simulink model "eVTOL_System"  (R2024b)
settings: Solver=FixedStepAuto  StartTime=0.0  StopTime=inf  RelTol=1e-3
undefined symbols (not defined in the file): airspeed, Battery, BCE12, BCE_Set_init, BMS_Controller_State, C, Cell10_P, Cell11_P, Cell12_P, Cell13_P, Cell14_P, Cell15_P, Cell16_P, Cell17_P, Cell18_P, Cell19_P, Cell1_N, Cell1_P, Cell20_P, Cell21_P, Cell22_P, Cell23_P, Cell24_P, Cell2_P, Cell3_P, Cell4_P, Cell5_P, Cell6_P, Cell7_P, Cell8_P, Cell9_P, Charging_State, CityMission, control, controlParams, ControlSampleTime, CriticalTiltAngle, currentFactor, CV_Gain, ddx, ddy, ddz, Device_01, Device_02, DiscIntNeverNeededParam, dx, dy, dz, Earth, env, F, F28379D_ADC_MaxCount, F28379D_ADC_Vmax, FixedWingMission, flightState, Foc_Ki_IxTcpu, Foc_Ki_S, Foc_Kp_I, Foc_Kp_S, fractalcoef ... (+68)
libraries: fl_lib x1115, nesl_utility x617, slrealtimeethercatlib x217, simulink x130, canmsglib x101, speedgoatlib_IO611_obsolete x91, slpidlib x49, mcbcontrolslib x44, slrealtimeutilitieslib x35, speedgoatlib_hdlCoder_IO3xx x31, dspstat3 x24, mcbpositiondecoderlib x12
(part 5 of 31)

== system eVTOL_System/Motor Drive/Controller1/Controller_MIL ==
  Iab : Inport
  QAE_MIL_fbk : Inport  Port=2
  EnablePWM : Inport  Port=3
  Closed_Loop_FOC : Inport  Port=4
  Speed_CMD_RPM : Inport  Port=5
  Controller_Parameters : Inport  Port=6
  Bus Creator : BusCreator  Inputs=5
  Bus Selector : BusSelector  OutputSignals=Ia_offset,Ib_offset,Kp_S,Ki_S,Kp_I,Ki_IxTcpu
  Constant : Constant  Value=0  OutDataTypeStr=single  SampleTime=Ts_CPU
  Constant4 : Constant
  Data Type Conversion : DataTypeConversion  SaturateOnIntegerOverflow=off  RndMeth=Floor
  Data Type Conversion1 : DataTypeConversion  OutDataTypeStr=double  SaturateOnIntegerOverflow=off  RndMeth=Floor
  Data Type Conversion2 : DataTypeConversion  OutDataTypeStr=boolean  SaturateOnIntegerOverflow=off  RndMeth=Floor
  Data Type Conversion4 : DataTypeConversion  OutDataTypeStr=boolean  SaturateOnIntegerOverflow=off  RndMeth=Floor
  Data Type Conversion6 : DataTypeConversion  OutDataTypeStr=uint16  RndMeth=Simplest  SaturateOnIntegerOverflow=off
  F28379D ADC : Subsystem
  F28379D Firmware : Subsystem
  IO334 DAC : Subsystem
  Mux : Mux  Inputs=3
  PWM Generation : pwm_cpulib/PWM Generation  f_FPGA=f_FPGA  n_channels=3  sel_scaling=CPU  protection_param=A/B are forced off when A/B are on.  deadband_sec=0  natural_update=At period starts  delay=0  trigger_duration_sec=[1e-6]  trigger_period_start=off  trigger_half_of_the_period=off  trigger_a_on=off  trigger_a_off=off  trigger_b_on=off  trigger_b_off=off  bit_width_pwm_gen=24  invert_a=off  invert_b=off  invert_c=off  showPhaseInput=off
      settings: SourceProductName=PWM CPU Library
  PWM Periods : Constant  Value=[1/PWM_frequency 1/PWM_frequency 1/PWM_frequency]  OutDataTypeStr=double  SampleTime=-1
  Rate Transition1 : RateTransition  OutPortSampleTime=Ts_speed
  Rate Transition12 : RateTransition  OutPortSampleTime=Ts_UI
  Rate Transition{2,4..9} (7 alike) : RateTransition  OutPortSampleTime=Ts_CPU
  Rate Transition3 : RateTransition  OutPortSampleTime=Ts_speed
  bias1 : Constant  OutDataTypeStr=boolean  SampleTime=Ts_CPU
  bias3 : Constant  Value=0  OutDataTypeStr=boolean  SampleTime=Ts_CPU
  Simu_config : Outport
  Controller_fbk : Outport  Port=2
  wires:
  bias1/1 -> Bus Creator/1  "PCIe_RC_or_TTL"
  Bus Creator/1 -> Simu_config/1
  Constant4/1 -> Data Type Conversion6/1
  Data Type Conversion/1 -> Bus Creator/4  "PCIe_PWM_Enable"
  Iab/1 -> IO334 DAC/1(Iab)
  IO334 DAC/1(Iab_IO334DAC) -> F28379D ADC/1(Iab_IO334V)  "IabV"
  F28379D ADC/1(Ia_ADC) -> F28379D Firmware/1(Ia_ADC)
  F28379D ADC/2(Ib_ADC) -> F28379D Firmware/2(Ib_ADC)
  QAE_MIL_fbk/1 -> F28379D Firmware/5(QEP_Position_Count)
  Data Type Conversion6/1 -> F28379D Firmware/6(QEP_Index_Latch)
  Bus Selector/3 -> Rate Transition3/1  "<Kp_S>"
  F28379D Firmware/2(PWM_Enable) -> Data Type Conversion/1
  Data Type Conversion2/1 -> F28379D Firmware/11(EnablePWM)
  Data Type Conversion4/1 -> F28379D Firmware/10(EnClosedLoop)
  Bus Selector/4 -> Rate Transition1/1  "<Ki_S>"
  Closed_Loop_FOC/1 -> Rate Transition4/1
  Controller_Parameters/1 -> Bus Selector/1
  Bus Selector/1 -> Rate Transition5/1  "<Ia_offset>"
  Bus Selector/2 -> Rate Transition6/1  "<Ib_offset>"
  Bus Selector/5 -> Rate Transition8/1  "<Kp_I>"
  Bus Selector/6 -> Rate Transition9/1  "<Ki_IxTcpu>"
  EnablePWM/1 -> Rate Transition7/1
  Mux/1 -> Rate Transition12/1
  F28379D Firmware/3(Fbk_CAN) -> Mux/1
  Speed_CMD_RPM/1 -> Rate Transition2/1
  Rate Transition3/1 -> F28379D Firmware/8(Kp_S)
  Rate Transition1/1 -> F28379D Firmware/9(Ki_S)
  Rate Transition5/1 -> F28379D Firmware/3(IaOffset)
  Rate Transition6/1 -> F28379D Firmware/4(IbOffset)
  Rate Transition4/1 -> Data Type Conversion4/1
  Rate Transition7/1 -> Data Type Conversion2/1
  Rate Transition8/1 -> F28379D Firmware/12(Kp_i)
  Rate Transition9/1 -> F28379D Firmware/13(Ki_ixTcpu)
  Rate Transition12/1 -> Controller_fbk/1
  Constant/1 -> Mux/3
  Rate Transition2/1 -> F28379D Firmware/7(SpdCmdRPM), Mux/2
  bias3/1 -> Bus Creator/5  "PCIe_Protocol"
  PWM Periods/1 -> PWM Generation/1
  PWM Generation/1 -> Bus Creator/2  "PCIe_PWM_Config"
  PWM Generation/2 -> Bus Creator/3  "PCIe_PWM_Runtime"
  Data Type Conversion1/1 -> PWM Generation/2
  F28379D Firmware/1(ModWave) -> Data Type Conversion1/1

== system eVTOL_System/Motor Drive/Controller2/Controller_MIL ==
  Iab : Inport
  QAE_MIL_fbk : Inport  Port=2
  EnablePWM : Inport  Port=3
  Closed_Loop_FOC : Inport  Port=4
  Speed_CMD_RPM : Inport  Port=5
  Controller_Parameters : Inport  Port=6
  Bus Creator : BusCreator  Inputs=5
  Bus Selector : BusSelector  OutputSignals=Ia_offset,Ib_offset,Kp_S,Ki_S,Kp_I,Ki_IxTcpu
  Constant : Constant  Value=0  OutDataTypeStr=single  SampleTime=Ts_CPU
  Constant4 : Constant
  Data Type Conversion : DataTypeConversion  SaturateOnIntegerOverflow=off  RndMeth=Floor
  Data Type Conversion1 : DataTypeConversion  OutDataTypeStr=double  SaturateOnIntegerOverflow=off  RndMeth=Floor
  Data Type Conversion2 : DataTypeConversion  OutDataTypeStr=boolean  SaturateOnIntegerOverflow=off  RndMeth=Floor
  Data Type Conversion4 : DataTypeConversion  OutDataTypeStr=boolean  SaturateOnIntegerOverflow=off  RndMeth=Floor
  Data Type Conversion6 : DataTypeConversion  OutDataTypeStr=uint16  RndMeth=Simplest  SaturateOnIntegerOverflow=off
  F28379D ADC : Subsystem
  F28379D Firmware : Subsystem
  IO334 DAC : Subsystem
  Mux : Mux  Inputs=3
  PWM Generation : pwm_cpulib/PWM Generation  f_FPGA=f_FPGA  n_channels=3  sel_scaling=CPU  protection_param=A/B are forced off when A/B are on.  deadband_sec=0  natural_update=At period starts  delay=0  trigger_duration_sec=[1e-6]  trigger_period_start=off  trigger_half_of_the_period=off  trigger_a_on=off  trigger_a_off=off  trigger_b_on=off  trigger_b_off=off  bit_width_pwm_gen=24  invert_a=off  invert_b=off  invert_c=off  showPhaseInput=off
      settings: SourceProductName=PWM CPU Library
  PWM Periods : Constant  Value=[1/PWM_frequency 1/PWM_frequency 1/PWM_frequency]  OutDataTypeStr=double  SampleTime=-1
  Rate Transition1 : RateTransition  OutPortSampleTime=Ts_speed
  Rate Transition12 : RateTransition  OutPortSampleTime=Ts_UI
  Rate Transition{2,4..9} (7 alike) : RateTransition  OutPortSampleTime=Ts_CPU
  Rate Transition3 : RateTransition  OutPortSampleTime=Ts_speed
  bias1 : Constant  OutDataTypeStr=boolean  SampleTime=Ts_CPU
  bias3 : Constant  Value=0  OutDataTypeStr=boolean  SampleTime=Ts_CPU
  Simu_config : Outport
  Controller_fbk : Outport  Port=2
  wires:
  bias1/1 -> Bus Creator/1  "PCIe_RC_or_TTL"
  Bus Creator/1 -> Simu_config/1
  Constant4/1 -> Data Type Conversion6/1
  Data Type Conversion/1 -> Bus Creator/4  "PCIe_PWM_Enable"
  Iab/1 -> IO334 DAC/1(Iab)
  IO334 DAC/1(Iab_IO334DAC) -> F28379D ADC/1(Iab_IO334V)  "IabV"
  F28379D ADC/1(Ia_ADC) -> F28379D Firmware/1(Ia_ADC)
  F28379D ADC/2(Ib_ADC) -> F28379D Firmware/2(Ib_ADC)
  QAE_MIL_fbk/1 -> F28379D Firmware/5(QEP_Position_Count)
  Data Type Conversion6/1 -> F28379D Firmware/6(QEP_Index_Latch)
  Bus Selector/3 -> Rate Transition3/1  "<Kp_S>"
  F28379D Firmware/2(PWM_Enable) -> Data Type Conversion/1
  Data Type Conversion2/1 -> F28379D Firmware/11(EnablePWM)
  Data Type Conversion4/1 -> F28379D Firmware/10(EnClosedLoop)
  Bus Selector/4 -> Rate Transition1/1  "<Ki_S>"
  Closed_Loop_FOC/1 -> Rate Transition4/1
  Controller_Parameters/1 -> Bus Selector/1
  Bus Selector/1 -> Rate Transition5/1  "<Ia_offset>"
  Bus Selector/2 -> Rate Transition6/1  "<Ib_offset>"
  Bus Selector/5 -> Rate Transition8/1  "<Kp_I>"
  Bus Selector/6 -> Rate Transition9/1  "<Ki_IxTcpu>"
  EnablePWM/1 -> Rate Transition7/1
  Mux/1 -> Rate Transition12/1
  F28379D Firmware/3(Fbk_CAN) -> Mux/1
  Speed_CMD_RPM/1 -> Rate Transition2/1
  Rate Transition3/1 -> F28379D Firmware/8(Kp_S)
  Rate Transition1/1 -> F28379D Firmware/9(Ki_S)
  Rate Transition5/1 -> F28379D Firmware/3(IaOffset)
  Rate Transition6/1 -> F28379D Firmware/4(IbOffset)
  Rate Transition4/1 -> Data Type Conversion4/1
  Rate Transition7/1 -> Data Type Conversion2/1
  Rate Transition8/1 -> F28379D Firmware/12(Kp_i)
  Rate Transition9/1 -> F28379D Firmware/13(Ki_ixTcpu)
  Rate Transition12/1 -> Controller_fbk/1
  Constant/1 -> Mux/3
  Rate Transition2/1 -> F28379D Firmware/7(SpdCmdRPM), Mux/2
  bias3/1 -> Bus Creator/5  "PCIe_Protocol"
  PWM Periods/1 -> PWM Generation/1
  PWM Generation/1 -> Bus Creator/2  "PCIe_PWM_Config"
  PWM Generation/2 -> Bus Creator/3  "PCIe_PWM_Runtime"
  Data Type Conversion1/1 -> PWM Generation/2
  F28379D Firmware/1(ModWave) -> Data Type Conversion1/1

== system eVTOL_System/Motor Drive/Controller3/Controller_MIL ==
  Iab : Inport
  QAE_MIL_fbk : Inport  Port=2
  EnablePWM : Inport  Port=3
  Closed_Loop_FOC : Inport  Port=4
  Speed_CMD_RPM : Inport  Port=5
  Controller_Parameters : Inport  Port=6
  Bus Creator : BusCreator  Inputs=5
  Bus Selector : BusSelector  OutputSignals=Ia_offset,Ib_offset,Kp_S,Ki_S,Kp_I,Ki_IxTcpu
  Constant : Constant  Value=0  OutDataTypeStr=single  SampleTime=Ts_CPU
  Constant4 : Constant
  Data Type Conversion : DataTypeConversion  SaturateOnIntegerOverflow=off  RndMeth=Floor
  Data Type Conversion1 : DataTypeConversion  OutDataTypeStr=double  SaturateOnIntegerOverflow=off  RndMeth=Floor
  Data Type Conversion2 : DataTypeConversion  OutDataTypeStr=boolean  SaturateOnIntegerOverflow=off  RndMeth=Floor
  Data Type Conversion4 : DataTypeConversion  OutDataTypeStr=boolean  SaturateOnIntegerOverflow=off  RndMeth=Floor
  Data Type Conversion6 : DataTypeConversion  OutDataTypeStr=uint16  RndMeth=Simplest  SaturateOnIntegerOverflow=off
  F28379D ADC : Subsystem
  F28379D Firmware : Subsystem
  IO334 DAC : Subsystem
  Mux : Mux  Inputs=3
  PWM Generation : pwm_cpulib/PWM Generation  f_FPGA=f_FPGA  n_channels=3  sel_scaling=CPU  protection_param=A/B are forced off when A/B are on.  deadband_sec=0  natural_update=At period starts  delay=0  trigger_duration_sec=[1e-6]  trigger_period_start=off  trigger_half_of_the_period=off  trigger_a_on=off  trigger_a_off=off  trigger_b_on=off  trigger_b_off=off  bit_width_pwm_gen=24  invert_a=off  invert_b=off  invert_c=off  showPhaseInput=off
      settings: SourceProductName=PWM CPU Library
  PWM Periods : Constant  Value=[1/PWM_frequency 1/PWM_frequency 1/PWM_frequency]  OutDataTypeStr=double  SampleTime=-1
  Rate Transition1 : RateTransition  OutPortSampleTime=Ts_speed
  Rate Transition12 : RateTransition  OutPortSampleTime=Ts_UI
  Rate Transition{2,4..9} (7 alike) : RateTransition  OutPortSampleTime=Ts_CPU
  Rate Transition3 : RateTransition  OutPortSampleTime=Ts_speed
  bias1 : Constant  OutDataTypeStr=boolean  SampleTime=Ts_CPU
  bias3 : Constant  Value=0  OutDataTypeStr=boolean  SampleTime=Ts_CPU
  Simu_config : Outport
  Controller_fbk : Outport  Port=2
  wires:
  bias1/1 -> Bus Creator/1  "PCIe_RC_or_TTL"
  Bus Creator/1 -> Simu_config/1
  Constant4/1 -> Data Type Conversion6/1
  Data Type Conversion/1 -> Bus Creator/4  "PCIe_PWM_Enable"
  Iab/1 -> IO334 DAC/1(Iab)
  IO334 DAC/1(Iab_IO334DAC) -> F28379D ADC/1(Iab_IO334V)  "IabV"
  F28379D ADC/1(Ia_ADC) -> F28379D Firmware/1(Ia_ADC)
  F28379D ADC/2(Ib_ADC) -> F28379D Firmware/2(Ib_ADC)
  QAE_MIL_fbk/1 -> F28379D Firmware/5(QEP_Position_Count)
  Data Type Conversion6/1 -> F28379D Firmware/6(QEP_Index_Latch)
  Bus Selector/3 -> Rate Transition3/1  "<Kp_S>"
  F28379D Firmware/2(PWM_Enable) -> Data Type Conversion/1
  Data Type Conversion2/1 -> F28379D Firmware/11(EnablePWM)
  Data Type Conversion4/1 -> F28379D Firmware/10(EnClosedLoop)
  Bus Selector/4 -> Rate Transition1/1  "<Ki_S>"
  Closed_Loop_FOC/1 -> Rate Transition4/1
  Controller_Parameters/1 -> Bus Selector/1
  Bus Selector/1 -> Rate Transition5/1  "<Ia_offset>"
  Bus Selector/2 -> Rate Transition6/1  "<Ib_offset>"
  Bus Selector/5 -> Rate Transition8/1  "<Kp_I>"
  Bus Selector/6 -> Rate Transition9/1  "<Ki_IxTcpu>"
  EnablePWM/1 -> Rate Transition7/1
  Mux/1 -> Rate Transition12/1
  F28379D Firmware/3(Fbk_CAN) -> Mux/1
  Speed_CMD_RPM/1 -> Rate Transition2/1
  Rate Transition3/1 -> F28379D Firmware/8(Kp_S)
  Rate Transition1/1 -> F28379D Firmware/9(Ki_S)
  Rate Transition5/1 -> F28379D Firmware/3(IaOffset)
  Rate Transition6/1 -> F28379D Firmware/4(IbOffset)
  Rate Transition4/1 -> Data Type Conversion4/1
  Rate Transition7/1 -> Data Type Conversion2/1
  Rate Transition8/1 -> F28379D Firmware/12(Kp_i)
  Rate Transition9/1 -> F28379D Firmware/13(Ki_ixTcpu)
  Rate Transition12/1 -> Controller_fbk/1
  Constant/1 -> Mux/3
  Rate Transition2/1 -> F28379D Firmware/7(SpdCmdRPM), Mux/2
  bias3/1 -> Bus Creator/5  "PCIe_Protocol"
  PWM Periods/1 -> PWM Generation/1
  PWM Generation/1 -> Bus Creator/2  "PCIe_PWM_Config"
  PWM Generation/2 -> Bus Creator/3  "PCIe_PWM_Runtime"
  Data Type Conversion1/1 -> PWM Generation/2
  F28379D Firmware/1(ModWave) -> Data Type Conversion1/1

== system eVTOL_System/Motor Drive/Three-Phase PMSM Drive/PMSM and average inverter ==
  Simu_config : Inport
  V_dc : Inport  Port=2
  Fault : Inport  Port=3
  LdTrq/Spd : Inport  Port=4
  Bus Selector : BusSelector  OutputSignals=PCIe_PWM_Runtime
  Demux : Demux  Outputs=3
  Encoder Simulation : Subsystem
  Idc : Subsystem
  Ideal Inverter : Subsystem
  PMSM : Subsystem
  PMSM HDL Configuration1 : mcbhdlplantlib/PMSM Configuration  portConfig=Torque  Trq_N_mode=0  Ts=Ts_CPU  Pp=7  Rs=0.293  Ld=0.000279  Lq=0.000279  lambda_pm=0.005  J=8.35e-5  B=0.00535  f=0.0065
  Runtime to DC : Subsystem
  Selec Angle1 : Selector  InputPortWidth=14  IndexOptions=Index vector (dialog)  Indices=[10]  OutputSizes=1
  Terminator : Terminator
  Terminator1 : Terminator
  Terminator2 : Terminator
  Ia : Outport
  Ib : Outport  Port=2
  Ic : Outport  Port=3
  Motor_Spd : Outport  Port=4
  Motor_Angle : Outport  Port=5
  QAE_Pos_C : Outport  Port=6
  tag scope: Idc1=global
  wires:
  PMSM/4(RotorMechSpd) -> Motor_Spd/1
  Demux/2 -> Ib/1
  Selec Angle1/1 -> Motor_Angle/1, Encoder Simulation/1(Theta_m)
  Demux/3 -> Ic/1
  LdTrq/Spd/1 -> PMSM/3(LdTrq / Spd)
  PMSM/2(PhaseCurr) -> Demux/1
  Demux/1 -> Idc/1(In1), Ia/1
  Ideal Inverter/1(Vabc) -> PMSM/2(PhaseVolt abc)
  V_dc/1 -> Ideal Inverter/1(V_DC)
  Simu_config/1 -> Bus Selector/1
  Fault/1 -> Terminator/1
  Encoder Simulation/1(QEP_Position_Count) -> QAE_Pos_C/1
  PMSM/3(Torque) -> Terminator1/1
  PMSM/5(RotorElecAngle) -> Terminator2/1
  PMSM/1(Info) -> Selec Angle1/1
  Bus Selector/1 -> Runtime to DC/1(PWM_Runtime)  "<PCIe_PWM_Runtime>"
  Runtime to DC/1(Duty Cycle abc) -> Ideal Inverter/2(Duty Cycle abc)
  PMSM HDL Configuration1/1 -> PMSM/1(Config)
  Idc/1(Out1) -> [Idc1]

== system eVTOL_System/Motor Drive/Three-Phase PMSM Drive/PMSM and inverter with switching dynamics ==
  Simu_config : Inport
  V_dc : Inport  Port=2
  Fault : Inport  Port=3
  LdTrq/Spd : Inport  Port=4
  Bus Selector : BusSelector  OutputSignals=PCIe_RC_or_TTL,PCIe_PWM_Config,PCIe_PWM_Runtime,PCIe_PWM_Enable,PCIe_Protocol
  DAC Config : Subsystem
  Encoder Simulation : Subsystem
  Idc : Subsystem
  Motor Connection : Constant  OutDataTypeStr=boolean
  PMSM HDL Configuration : mcbhdlplantlib/PMSM Configuration  portConfig=Torque  Trq_N_mode=0  Ts=Ts_UI  Pp=Maxon_645604_Np  Rs=Maxon_645604_Rs  Ld=Maxon_645604_Ld  Lq=Maxon_645604_Lq  lambda_pm=Maxon_645604_lambda_pm  J=Maxon_645604_J  B=Maxon_645604_ViscousF*100  f=Maxon_645604_StaticF
  PMSM_3P2L_Inverter_Plant_TBR : Subsystem
      mask Display: disp('Plant Bitstream Block')
  Quadrature Encoder : quadrature_cpulib/Quadrature Encoder  FPGA_freq=f_FPGA  n_channels=[1]  sel_scaling=FPGA  useSpeed=off  usePosition=on  numOfSlots=Maxon_Mile_Nslits  sigAswitchOn=[180]  sigBswitchOff=[90]  sigBswitchOn=[270]  sigAdismissEn=off  sigAdismissSingle=on  sigAdismissHigh=on  sigBdismissEn=off  sigBdismissSingle=on  sigBdismissHigh=on
      settings: SourceProductName=Quadrature CPU Library
  Resolver Encoder : resolver_cpulib/Resolver Encoder  Ts=Ts_UI  ts_resolver=ts_FPGA_mdl  n_channels=1  sel_scaling=FPGA  useSpeed=on  usePosition=off  pole_pairs=1  gain_dynamic=off  gainVector=[1, 1, 1, 1]  offset_dynamic=off  offsetVector=[0, 0, 0, 0]  exct_freq=2  angle_offset=0  exct_amplitude=10  position_init_enb=off  rotor_position=90  int_exct_enb=on  exct_out_enb=on  phase_delay=0  time_step_delay=0  adcRange=2.5  dacRange=2.5
      settings: SourceProductName=Resolver CPU Library
  Terminator{21,32..34,40..41,45..46} (8 alike) : Terminator
  Ia : Outport
  Ib : Outport  Port=2
  Ic : Outport  Port=3
  Motor_Spd : Outport  Port=4
  Motor_Angle : Outport  Port=5
  QAE_Pos_C : Outport  Port=6
  tag scope: Idc1=global
  wires:
  PMSM_3P2L_Inverter_Plant_TBR/10(PCIe_Rsvl_excitation_neg) -> Terminator33/1
  DAC Config/1(I_DAC_gain) -> PMSM_3P2L_Inverter_Plant_TBR/13(PCIe_Iabc_DAC_gain)
  DAC Config/3(DAC_reset) -> PMSM_3P2L_Inverter_Plant_TBR/15(PCIe_DAC_reset)
  PMSM_3P2L_Inverter_Plant_TBR/7(PCIe_Motor_ElecAngle) -> Terminator21/1
  PMSM_3P2L_Inverter_Plant_TBR/12(PCIe_Rsvl_cos_neg) -> Terminator41/1
  PMSM_3P2L_Inverter_Plant_TBR/13(PCIe_Resolver_Out) -> Terminator40/1
  V_dc/1 -> PMSM_3P2L_Inverter_Plant_TBR/6(PCIe_V_dc)
  PMSM_3P2L_Inverter_Plant_TBR/8(PCIe_Motor_Trq) -> Terminator46/1
  Resolver Encoder/1 -> PMSM_3P2L_Inverter_Plant_TBR/12(PCIe_Resolver_Config)
  PMSM_3P2L_Inverter_Plant_TBR/4(PCIe_Idc) -> Terminator45/1
  Quadrature Encoder/1 -> PMSM_3P2L_Inverter_Plant_TBR/11(PCIe_QAE_Config)
  Motor Connection/1 -> PMSM_3P2L_Inverter_Plant_TBR/10(PCIe_Motor_Connection)
  PMSM_3P2L_Inverter_Plant_TBR/9(PCIe_Rsvl_excitation_pos) -> Terminator32/1
  Fault/1 -> PMSM_3P2L_Inverter_Plant_TBR/7(PCIe_Fault)
  PMSM_3P2L_Inverter_Plant_TBR/11(PCIe_Rsvl_sin_neg) -> Terminator34/1
  DAC Config/2(I_DAC_Current) -> PMSM_3P2L_Inverter_Plant_TBR/14(PCIe_Iabc_DAC_bias)
  PMSM HDL Configuration/1 -> PMSM_3P2L_Inverter_Plant_TBR/9(PCIe_Motor_Config)
  Simu_config/1 -> Bus Selector/1
  Bus Selector/4 -> PMSM_3P2L_Inverter_Plant_TBR/4(PCIe_PWM_Enable)  "<PCIe_PWM_Enable>"
  Bus Selector/5 -> PMSM_3P2L_Inverter_Plant_TBR/5(PCIe_Protocol)  "<PCIe_Protocol>"
  Bus Selector/1 -> PMSM_3P2L_Inverter_Plant_TBR/1(PCIe_RC_or_TTL)  "<PCIe_RC_or_TTL>"
  LdTrq/Spd/1 -> PMSM_3P2L_Inverter_Plant_TBR/8(PCIe_LdTrq/Spd)
  PMSM_3P2L_Inverter_Plant_TBR/3(PCIe_Ic) -> Ic/1
  PMSM_3P2L_Inverter_Plant_TBR/6(PCIe_Motor_Angle) -> Motor_Angle/1, Encoder Simulation/1(Theta_m)
  PMSM_3P2L_Inverter_Plant_TBR/5(PCIe_Motor_Spd) -> Motor_Spd/1
  PMSM_3P2L_Inverter_Plant_TBR/2(PCIe_Ib) -> Ib/1
  Encoder Simulation/1(QEP_Position_Count) -> QAE_Pos_C/1
  Bus Selector/3 -> PMSM_3P2L_Inverter_Plant_TBR/3(PCIe_PWM_Runtime)  "<PCIe_PWM_Runtime>"
  Bus Selector/2 -> PMSM_3P2L_Inverter_Plant_TBR/2(PCIe_PWM_Config)  "<PCIe_PWM_Config>"
  Idc/1(Out1) -> [Idc1]
  PMSM_3P2L_Inverter_Plant_TBR/1(PCIe_Ia) -> Idc/1(In1), Ia/1

== system eVTOL_System/Motor Drive/Three-Phase PMSM Drive1/PMSM and average inverter ==
  Simu_config : Inport
  V_dc : Inport  Port=2
  Fault : Inport  Port=3
  LdTrq/Spd : Inport  Port=4
  Bus Selector : BusSelector  OutputSignals=PCIe_PWM_Runtime
  Demux : Demux  Outputs=3
  Encoder Simulation : Subsystem
  Idc : Subsystem
  Ideal Inverter : Subsystem
  PMSM : Subsystem
  PMSM HDL Configuration5 : mcbhdlplantlib/PMSM Configuration  portConfig=Torque  Trq_N_mode=0  Ts=Ts_CPU  Pp=7  Rs=0.293  Ld=0.000279  Lq=0.000279  lambda_pm=0.005  J=8.35e-5  B=0.00535  f=0.0065
  Runtime to DC : Subsystem
  Selec Angle1 : Selector  InputPortWidth=14  IndexOptions=Index vector (dialog)  Indices=[10]  OutputSizes=1
  Terminator : Terminator
  Terminator1 : Terminator
  Terminator2 : Terminator
  Ia : Outport
  Ib : Outport  Port=2
  Ic : Outport  Port=3
  Motor_Spd : Outport  Port=4
  Motor_Angle : Outport  Port=5
  QAE_Pos_C : Outport  Port=6
  tag scope: Idc2=global
  wires:
  PMSM/4(RotorMechSpd) -> Motor_Spd/1
  Demux/2 -> Ib/1
  Selec Angle1/1 -> Motor_Angle/1, Encoder Simulation/1(Theta_m)
  Demux/3 -> Ic/1
  LdTrq/Spd/1 -> PMSM/3(LdTrq / Spd)
  PMSM/2(PhaseCurr) -> Demux/1
  Ideal Inverter/1(Vabc) -> PMSM/2(PhaseVolt abc)
  Simu_config/1 -> Bus Selector/1
  Fault/1 -> Terminator/1
  Encoder Simulation/1(QEP_Position_Count) -> QAE_Pos_C/1
  PMSM/3(Torque) -> Terminator1/1
  PMSM/5(RotorElecAngle) -> Terminator2/1
  PMSM/1(Info) -> Selec Angle1/1
  Bus Selector/1 -> Runtime to DC/1(PWM_Runtime)  "<PCIe_PWM_Runtime>"
  Runtime to DC/1(Duty Cycle abc) -> Ideal Inverter/2(Duty Cycle abc)
  V_dc/1 -> Ideal Inverter/1(V_DC)
  Demux/1 -> Idc/1(In1), Ia/1
  PMSM HDL Configuration5/1 -> PMSM/1(Config)
  Idc/1(Out1) -> [Idc2]

== system eVTOL_System/Motor Drive/Three-Phase PMSM Drive2/PMSM and average inverter ==
  Simu_config : Inport
  V_dc : Inport  Port=2
  Fault : Inport  Port=3
  LdTrq/Spd : Inport  Port=4
  Bus Selector : BusSelector  OutputSignals=PCIe_PWM_Runtime
  Demux : Demux  Outputs=3
  Encoder Simulation : Subsystem
  Idc : Subsystem
  Ideal Inverter : Subsystem
  PMSM : Subsystem
  PMSM HDL Configuration5 : mcbhdlplantlib/PMSM Configuration  portConfig=Torque  Trq_N_mode=0  Ts=Ts_CPU  Pp=7  Rs=0.293  Ld=0.000279  Lq=0.000279  lambda_pm=0.005  J=8.35e-5  B=0.00535  f=0.0065
  Runtime to DC : Subsystem
  Selec Angle1 : Selector  InputPortWidth=14  IndexOptions=Index vector (dialog)  Indices=[10]  OutputSizes=1
  Terminator : Terminator
  Terminator1 : Terminator
  Terminator2 : Terminator
  Ia : Outport
  Ib : Outport  Port=2
  Ic : Outport  Port=3
  Motor_Spd : Outport  Port=4
  Motor_Angle : Outport  Port=5
  QAE_Pos_C : Outport  Port=6
  tag scope: Idc3=global
  wires:
  PMSM/4(RotorMechSpd) -> Motor_Spd/1
  Demux/2 -> Ib/1
  Selec Angle1/1 -> Motor_Angle/1, Encoder Simulation/1(Theta_m)
  Demux/3 -> Ic/1
  LdTrq/Spd/1 -> PMSM/3(LdTrq / Spd)
  PMSM/2(PhaseCurr) -> Demux/1
  Ideal Inverter/1(Vabc) -> PMSM/2(PhaseVolt abc)
  Simu_config/1 -> Bus Selector/1
  Fault/1 -> Terminator/1
  Encoder Simulation/1(QEP_Position_Count) -> QAE_Pos_C/1
  PMSM/3(Torque) -> Terminator1/1
  PMSM/5(RotorElecAngle) -> Terminator2/1
  PMSM/1(Info) -> Selec Angle1/1
  Bus Selector/1 -> Runtime to DC/1(PWM_Runtime)  "<PCIe_PWM_Runtime>"
  Runtime to DC/1(Duty Cycle abc) -> Ideal Inverter/2(Duty Cycle abc)
  V_dc/1 -> Ideal Inverter/1(V_DC)
  Demux/1 -> Idc/1(In1), Ia/1
  PMSM HDL Configuration5/1 -> PMSM/1(Config)
  Idc/1(Out1) -> [Idc3]

== system eVTOL_System/Motor Drive/Three-Phase PMSM Drive3/PMSM and average inverter ==
  Simu_config : Inport
  V_dc : Inport  Port=2
  Fault : Inport  Port=3
  LdTrq/Spd : Inport  Port=4
  Bus Selector : BusSelector  OutputSignals=PCIe_PWM_Runtime
  Demux : Demux  Outputs=3
  Encoder Simulation : Subsystem
  Idc : Subsystem
  Ideal Inverter : Subsystem
  PMSM : Subsystem
  PMSM HDL Configuration5 : mcbhdlplantlib/PMSM Configuration  portConfig=Torque  Trq_N_mode=0  Ts=Ts_CPU  Pp=7  Rs=0.293  Ld=0.000279  Lq=0.000279  lambda_pm=0.005  J=8.35e-5  B=0.00535  f=0.0065
  Runtime to DC : Subsystem
  Selec Angle1 : Selector  InputPortWidth=14  IndexOptions=Index vector (dialog)  Indices=[10]  OutputSizes=1
  Terminator : Terminator
  Terminator1 : Terminator
  Terminator2 : Terminator
  Ia : Outport
  Ib : Outport  Port=2
  Ic : Outport  Port=3
  Motor_Spd : Outport  Port=4
  Motor_Angle : Outport  Port=5
  QAE_Pos_C : Outport  Port=6
  tag scope: Idc4=global
  wires:
  PMSM/4(RotorMechSpd) -> Motor_Spd/1
  Demux/2 -> Ib/1
  Selec Angle1/1 -> Motor_Angle/1, Encoder Simulation/1(Theta_m)
  Demux/3 -> Ic/1
  LdTrq/Spd/1 -> PMSM/3(LdTrq / Spd)
  PMSM/2(PhaseCurr) -> Demux/1
  Ideal Inverter/1(Vabc) -> PMSM/2(PhaseVolt abc)
  Simu_config/1 -> Bus Selector/1
  Fault/1 -> Terminator/1
  Encoder Simulation/1(QEP_Position_Count) -> QAE_Pos_C/1
  PMSM/3(Torque) -> Terminator1/1
  PMSM/5(RotorElecAngle) -> Terminator2/1
  PMSM/1(Info) -> Selec Angle1/1
  Bus Selector/1 -> Runtime to DC/1(PWM_Runtime)  "<PCIe_PWM_Runtime>"
  Runtime to DC/1(Duty Cycle abc) -> Ideal Inverter/2(Duty Cycle abc)
  V_dc/1 -> Ideal Inverter/1(V_DC)
  Demux/1 -> Idc/1(In1), Ia/1
  PMSM HDL Configuration5/1 -> PMSM/1(Config)
  Idc/1(Out1) -> [Idc4]

== system eVTOL_System/Visualization/Photorealistic/PhotorealisticHIL ==
  UAVState : Inport
  Bus Creator : BusCreator  Inputs=6
  Bus Selector : BusSelector  OutputSignals=Euler,Xe
  Byte Pack : etargetslib/Byte Pack  datatypes={'double'}  byteAlign=1
  Byte Pack1 : etargetslib/Byte Pack  datatypes={'double'}  byteAlign=1
  Demux : Demux  Outputs=3
  Demux1 : Demux  Outputs=3
  Prepare UAV Data : Subsystem
  Send : slrealtimeiplib/UDP Send  useHostTargetConn=on  toAddress=172.16.20.80  toPort=25002  sampleTime=-1  enableMessage=off  ipAddress=172.16.19.29  localPort=-1
  Send1 : slrealtimeiplib/UDP Send  useHostTargetConn=on  toAddress=172.16.20.80  toPort=25003  sampleTime=-1  enableMessage=off  ipAddress=172.16.19.29  localPort=-1
  Width1 : Width
  Width2 : Width
  wires:
  Byte Pack/1 -> Width1/1, Send/1
  Prepare UAV Data/1(Translation) -> Byte Pack/1
  Demux1/1 -> Bus Creator/4  "x"
  Byte Pack1/1 -> Send1/1, Width2/1
  Prepare UAV Data/2(Rotation) -> Byte Pack1/1
  Width2/1 -> Send1/2
  Bus Selector/1 -> Demux/1  "<Euler>"
  Bus Creator/1 -> Prepare UAV Data/1(UAVState)
  Demux/1 -> Bus Creator/1  "roll"
  Width1/1 -> Send/2
  Demux/3 -> Bus Creator/3  "yaw"
  Demux1/3 -> Bus Creator/6  "z"
  Demux1/2 -> Bus Creator/5  "y"
  UAVState/1 -> Bus Selector/1
  Demux/2 -> Bus Creator/2  "pitch"
  Bus Selector/2 -> Demux1/1  "<Xe>"

== system eVTOL_System/Visualization/Photorealistic/PhotorealisticMIL ==
  UAVState : Inport
  Bus Creator : BusCreator  Inputs=6
  Bus Selector : BusSelector  OutputSignals=Euler,Xe
  Byte Pack : etargetslib/Byte Pack  datatypes={'double'}  byteAlign=1
  Byte Pack1 : etargetslib/Byte Pack  datatypes={'double'}  byteAlign=1
  Demux : Demux  Outputs=3
  Demux1 : Demux  Outputs=3
  Prepare UAV Data : Subsystem
  Send : slrealtimeiplib/UDP Send  useHostTargetConn=on  toAddress=172.16.20.80  toPort=25002  sampleTime=-1  enableMessage=off  ipAddress=172.16.19.29  localPort=-1
  Send1 : slrealtimeiplib/UDP Send  useHostTargetConn=on  toAddress=172.16.20.80  toPort=25003  sampleTime=-1  enableMessage=off  ipAddress=172.16.19.29  localPort=-1
  Width1 : Width
  Width2 : Width
  wires:
  Byte Pack/1 -> Width1/1, Send/1
  Prepare UAV Data/1(Translation) -> Byte Pack/1
  Demux1/1 -> Bus Creator/4  "x"
  Byte Pack1/1 -> Send1/1, Width2/1
  Prepare UAV Data/2(Rotation) -> Byte Pack1/1
  Width2/1 -> Send1/2
  Bus Selector/1 -> Demux/1  "<Euler>"
  Bus Creator/1 -> Prepare UAV Data/1(UAVState)
  Demux/1 -> Bus Creator/1  "roll"
  Width1/1 -> Send/2
  Demux/3 -> Bus Creator/3  "yaw"
  Demux1/3 -> Bus Creator/6  "z"
  Demux1/2 -> Bus Creator/5  "y"
  UAVState/1 -> Bus Selector/1
  Demux/2 -> Bus Creator/2  "pitch"
  Bus Selector/2 -> Demux1/1  "<Xe>"

== system eVTOL_System/Visualization/Visualization/VisualizationHIL ==
  UAVState : Inport
  Bus Selector : BusSelector  OutputSignals=Xe,q,RotorParameters.Rotor A,RotorParameters.Rotor B
  Byte Pack : etargetslib/Byte Pack  datatypes={'double'}  byteAlign=1
  Demux : Demux  Outputs=3
  Demux1 : Demux
  Mux : Mux  Inputs=9
  Send : slrealtimeiplib/UDP Send  useHostTargetConn=on  toAddress=172.16.19.25  toPort=25002  sampleTime=-1  enableMessage=off  ipAddress=172.16.19.29  localPort=-1
  Width1 : Width
  wires:
  Mux/1 -> Byte Pack/1
  Bus Selector/4 -> Mux/9  "<Rotor B>"
  Width1/1 -> Send/2
  UAVState/1 -> Bus Selector/1
  Byte Pack/1 -> Width1/1, Send/1
  Bus Selector/2 -> Demux1/1  "<q>"
  Demux/2 -> Mux/2
  Demux1/4 -> Mux/7
  Demux1/3 -> Mux/6
  Demux1/2 -> Mux/5
  Bus Selector/3 -> Mux/8  "<Rotor A>"
  Demux/1 -> Mux/1
  Demux1/1 -> Mux/4
  Demux/3 -> Mux/3
  Bus Selector/1 -> Demux/1  "<Xe>"

== system eVTOL_System/Visualization/Visualization/VisualizationMIL ==
  UAVState : Inport
  Bus Selector : BusSelector  OutputSignals=Xe,q,RotorParameters.Rotor A,RotorParameters.Rotor B
  Gain : Gain  Gain=0
  Subsystem : Subsystem
  Trajectory : uavutilslib/UAV Animation  NumUAV=1  DynamicUAVConfig=off  UAVType=FixedWing  UAVSize=6  UAVColor=[1 0 0]  UAVTrajectoryAlpha=1  InertialZDirection=Down  RotationFormat=Quaternion  DrawMarkers=off  SampleTime=0.1
  wires:
  Bus Selector/3 -> Subsystem/3(RotorA)  "<Rotor A>"
  UAVState/1 -> Bus Selector/1
  Bus Selector/2 -> Subsystem/2(<q>), Trajectory/2  "<q>"
  Bus Selector/4 -> Subsystem/4(RotorB)  "<Rotor B>"
  Bus Selector/1 -> Gain/1, Trajectory/1  "<Xe>"
  Gain/1 -> Subsystem/1(<Xe>)

== system eVTOL_System/Battery System/BMS/HIL/Cell Monitoring Unit ==
  Bal_Cmd_Controller : Inport
  Sensor_Values : Inport  Port=2
  Balancing_Circuit3 : Subsystem  Commented=on
  Balancing_Circuit4 : Subsystem  Commented=on
  CMU1 : Subsystem
  CMU2 : Subsystem
  Cells1 : PMIOPort  Side=Left
  Cells2 : PMIOPort  Port=2  Side=Left
  Sensor Values : Outport
  tag scope: Balancing_Currents1=global, Balancing_Currents2=global
  wires:
  Sensor_Values/1 -> Sensor Values/1
  Bal_Cmd_Controller/1 -> CMU1/1(Bal_Cmd_Controller), CMU2/1(Bal_Cmd_Controller)  "Bal_Cmd"
  CMU1/1(Balancing_Currents) -> [Balancing_Currents1]
  CMU2/1(Balancing_Currents) -> [Balancing_Currents2]
  connections:
  Cells1/RConn1 -- CMU1/LConn1
  Cells2/RConn1 -- CMU2/LConn1

== system eVTOL_System/Battery System/BMS/HIL/Controller_100Cells ==
  Sensor_Values : Inport  OutDataTypeStr=Bus: Sensor_Values  BusOutputAsStruct=on
  State_Request : Inport  Port=2  OutDataTypeStr=Enum: SRE  PortDimensions=1
  CAN & LIN Setup : speedgoatlib_IO611_obsolete/CAN & LIN Setup  id=1  drvLtr=C:  PCISlot=-1  port1=CAN (HS/LS)  port2=CAN (HS/LS)  port3=Disable  port4=Disable  opModeCAN1=Highspeed (HS)  bdrCAN1=1 MBaud  usrBdrCAN1=[5, 1, 13, 2]  bdrFD1=5 MBaud  usrBdrFD1=[2, 1, 5, 2, 75, 5000]  stdAccMaskCAN1=[0, 0]  extAccMaskCAN1=[0, 0]  opModeCAN2=Highspeed (HS)  bdrCAN2=1 MBaud  usrBdrCAN2=[5, 1, 13, 2]  bdrFD2=5 MBaud  usrBdrFD2=[2, 1, 5, 2, 75, 5000]  stdAccMaskCAN2=[0, 0]  extAccMaskCAN2=[0, 0]  initStruct=[]  termStruct=[]  opModeLIN3=Master  bdrLIN3=19200  opModeLIN4=Master  bdrLIN4=19200  protl=IO611  qtyMod=1  chNo=[1, 2, 3, 4]  ptTypes=[1, 1, 2, 2]  isProtlFD=[0, 0]  protlHelpIdx=[0, 1, 0, 1]  isFDMod=1
      settings: SourceProductName=IO611
  Constant10 : Constant  Value=uint8(SRE.Charging)
  Constant8 : Constant  Value=uint8(SRE.Standby)
  Constant9 : Constant  Value=uint8(SRE.Flying)
  Multiport Switch : MultiPortSwitch  DataPortOrder=Specify indices  DataPortIndices={SRE.Standby, SRE.Flying, SRE.Charging}  SaturateOnIntegerOverflow=off  InputSameDT=off
  PLANT-Rx : Subsystem  TreatAsAtomicUnit=on
  PLANT-Tx : Subsystem
  Rate Transition : RateTransition  InitialCondition=struct('OverCurrent',0,'HighTemp',0,'LowTemp',0,'OverVolt',0,'UnderVolt',0)  OutPortSampleTime=ts_controller
  Rate Transition1 : RateTransition  InitialCondition=Charging_State.Init  OutPortSampleTime=ts_controller
  Rate Transition2 : RateTransition  InitialCondition=BMS_Controller_State.BMS_Idle  OutPortSampleTime=ts_controller
  Rate Transition3 : RateTransition  InitialCondition=[0, 0, 0]  OutPortSampleTime=ts_controller
  Rate Transition4 : RateTransition  InitialCondition=-100  OutPortSampleTime=ts_controller
  Rate Transition5 : RateTransition  InitialCondition=40  OutPortSampleTime=ts_controller
  Rate Transition6 : RateTransition  OutPortSampleTime=ts_controller
  Rate Transition7 : RateTransition  OutPortSampleTime=ts_controller
  BMS_Faults : Outport
  Charging_State : Outport  Port=2
  BMS_State : Outport  Port=3
  SOC : Outport  Port=4
  Discharge_Current_Limit : Outport  Port=5
  Charge_Current_Limit : Outport  Port=6
  Charge_Current_Req : Outport  Port=7
  Bal_Cmd_76Cells : Outport  Port=8
  wires:
  Constant9/1 -> Multiport Switch/3
  Constant10/1 -> Multiport Switch/4
  Constant8/1 -> Multiport Switch/2
  State_Request/1 -> Multiport Switch/1
  PLANT-Rx/1(BMS_Faults) -> Rate Transition/1
  PLANT-Rx/7(Charge_Current_Req) -> Rate Transition6/1
  PLANT-Rx/6(Charge_Current_Limit) -> Rate Transition5/1
  PLANT-Rx/5(Discharge_Current_Limit) -> Rate Transition4/1
  PLANT-Rx/4(SOC) -> Rate Transition3/1
  PLANT-Rx/3(BMS_State) -> Rate Transition2/1
  PLANT-Rx/2(Charging_State) -> Rate Transition1/1
  Rate Transition/1 -> BMS_Faults/1  "Faults"
  Rate Transition1/1 -> Charging_State/1  "Charging_State"
  Rate Transition2/1 -> BMS_State/1  "BMS_State"
  Rate Transition3/1 -> SOC/1  "SOC"
  Rate Transition4/1 -> Discharge_Current_Limit/1  "Discharge_Current_Limit"
  Rate Transition5/1 -> Charge_Current_Limit/1  "Charge_Current_Limit"
  Rate Transition6/1 -> Charge_Current_Req/1  "Charge_Current_Req"
  Sensor_Values/1 -> PLANT-Tx/1(to_Controller)
  Multiport Switch/1 -> PLANT-Tx/2(to_Controller_SRE)  "SRE"
  Rate Transition7/1 -> Bal_Cmd_76Cells/1  "Bal_Cmd_76Cells"
  PLANT-Rx/8(Bal_Cmd_76Cells) -> Rate Transition7/1

== system eVTOL_System/Battery System/BMS/HIL/Controller_76Cells ==
  Sensor_Values : Inport  OutDataTypeStr=Bus: Sensor_Values  BusOutputAsStruct=on
  State_Request : Inport  Port=2  OutDataTypeStr=Enum: SRE  PortDimensions=1
  BMS State Machine : Subsystem
  Balancing Logic : Subsystem
  Constant : Constant
  Current Calculations : Subsystem
  SOC Calculation : Subsystem
  Faults : Outport
  Charging_State : Outport  Port=2
  BMS_Controller_State : Outport  Port=3
  SOC : Outport  Port=4
  Discharge_Current_Limit : Outport  Port=5
  Charge_Current_Limit : Outport  Port=6
  Charge_Current_Req : Outport  Port=7
  Bal_Cmd1 : Outport  Port=8
  wires:
  SOC Calculation/1(SOC) -> SOC/1
  Current Calculations/1(Discharge_Current_Limit) -> Discharge_Current_Limit/1, BMS State Machine/1(Discharge_Current_Limit)
  BMS State Machine/2(Faults) -> Faults/1
  BMS State Machine/1(Charge_Current_Req) -> Charge_Current_Req/1
  Sensor_Values/1 -> Balancing Logic/2(Sensor_Values), SOC Calculation/2(Sensor_Values), BMS State Machine/4(Sensor_Values), Current Calculations/1(BMS_Input)
  BMS State Machine/4(BMS_State) -> BMS_Controller_State/1, SOC Calculation/1(BMS_State), Balancing Logic/1(BMS_State)
  Current Calculations/2(Charge_Current_Limit) -> Charge_Current_Limit/1, BMS State Machine/2(Charge_Current_Limit)
  Balancing Logic/1(Bal_Cmd1) -> Bal_Cmd1/1  "Bal_Cmd1"
  State_Request/1 -> BMS State Machine/3(State_Request)
  Constant/1 -> BMS State Machine/5(Fault_Reset_Enable)
  BMS State Machine/3(Charging_State) -> Charging_State/1

== system eVTOL_System/Battery System/BMS/MIL/Cell Monitoring Unit ==
  Bal_Cmd_Controller : Inport
  Sensor_Values : Inport  Port=2
  Balancing_Circuit : Subsystem
  Balancing_Circuit1 : Subsystem
  Balancing_Circuit2 : Subsystem
  Delay : Delay  DelayLength=1
  Feedback Unit1 : UnitDelay  Commented=on  InitialCondition=struct('Cell_Voltages',3.6*ones(1, Ns_Module*NumModules),'Cell_Temperatures',293.15*ones(1,Ns_Module*NumModules),'Pack_Current',0,'Pack_Voltage',3.6*Ns_Module*NumModules)  SampleTime=-1  HasFrameUpgradeWarning=on
  Rate Transition1 : RateTransition  InitialCondition=zeros(1,Ns_Module)  OutPortSampleTime=ts_system
  Cells : PMIOPort  Side=Left
  Cells1 : PMIOPort  Port=2  Side=Left
  Cells2 : PMIOPort  Port=3  Side=Left
  Sensor Values : Outport
  tag scope: Balancing_Currents1=global, Balancing_Currents2=global, Balancing_Currents=global
  wires:
  Sensor_Values/1 -> Delay/1
  Bal_Cmd_Controller/1 -> Rate Transition1/1
  Rate Transition1/1 -> Balancing_Circuit1/1(Bal_Cmd_Controller), Balancing_Circuit2/1(Bal_Cmd_Controller), Balancing_Circuit/1(Bal_Cmd_Controller)
  Balancing_Circuit/1(Balancing_Currents) -> [Balancing_Currents]
  Delay/1 -> Sensor Values/1
  Balancing_Circuit1/1(Balancing_Currents) -> [Balancing_Currents1]
  Balancing_Circuit2/1(Balancing_Currents) -> [Balancing_Currents2]
  connections:
  Balancing_Circuit/LConn1 -- Cells/RConn1
  Cells1/RConn1 -- Balancing_Circuit1/LConn1
  Balancing_Circuit2/LConn1 -- Cells2/RConn1

== system eVTOL_System/Battery System/BMS/MIL/Controller ==
  Sensor_Values : Inport  OutDataTypeStr=Bus: Sensor_Values  BusOutputAsStruct=on
  State_Request : Inport  Port=2  OutDataTypeStr=Enum: SRE  PortDimensions=1
  BMS State Machine : Subsystem
  Balancing Logic : Subsystem
  Constant : Constant
  Current Calculations : Subsystem
  SOC Calculation : Subsystem
  Faults : Outport
  Charging_State : Outport  Port=2
  BMS_Controller_State : Outport  Port=3
  SOC : Outport  Port=4
  Discharge_Current_Limit : Outport  Port=5
  Charge_Current_Limit : Outport  Port=6
  Charge_Current_Req : Outport  Port=7
  Bal_Cmd : Outport  Port=8
  wires:
  SOC Calculation/1(SOC) -> SOC/1
  Current Calculations/1(Discharge_Current_Limit) -> Discharge_Current_Limit/1, BMS State Machine/1(Discharge_Current_Limit)
  BMS State Machine/2(Faults) -> Faults/1
  BMS State Machine/1(Charge_Current_Req) -> Charge_Current_Req/1
  Sensor_Values/1 -> Balancing Logic/2(Sensor_Values), SOC Calculation/2(Sensor_Values), BMS State Machine/4(Sensor_Values), Current Calculations/1(BMS_Input)
  BMS State Machine/4(BMS_State) -> BMS_Controller_State/1, SOC Calculation/1(BMS_State), Balancing Logic/1(BMS_State)
  Current Calculations/2(Charge_Current_Limit) -> Charge_Current_Limit/1, BMS State Machine/2(Charge_Current_Limit)
  Balancing Logic/1(Bal_Cmd) -> Bal_Cmd/1  "Bal_Cmd"
  State_Request/1 -> BMS State Machine/3(State_Request)
  Constant/1 -> BMS State Machine/5(Fault_Reset_Enable)
  BMS State Machine/3(Charging_State) -> Charging_State/1
